simulink model "DB_HFI_sim"  (R2017a)
settings: Solver=ode45  StartTime=0.0  StopTime=20  FixedStep=0.5e-4  MaxStep=1e-4  RelTol=2.8e-10  AbsTol=eps  EnableMultiTasking=on
InitFcn:
  | %makec
model workspace: external: MAT-File C:\Users\Bench_39\Documents\MATLAB\DBDTFC_SelfSensing\ws.mat (data not in the file)
values from neighbouring files (symbols this model uses):
  bp = 2.2e-4    (= 0.00022)    [IPMSM_param.m]    (also in ws.mat)
  j = [0, -1; 1, 0]    [init.m]    (also in ws.mat = [0  -1; 1  0])
  Jp = 3.2e-4    (= 0.00032)    [IPMSM_param.m]    (also in ws.mat)
  lambda_pm = 0.13    [IPMSM_param.m]    (also in ws.mat)
  Ld = 8e-3    (= 0.008)    [IPMSM_param.m]    (also in ws.mat)
  Ldq = [Ld Lqd ;  Lqd Lq]    [IPMSM_param.m]    (also in ws.mat = [0.008  0; 0  0.02])
  Lq = 20e-3    (= 0.02)    [IPMSM_param.m]    (also in ws.mat)
  p = 2    [IPMSM_param.m]    (also in ws.mat)
  Rs = 1.35    [IPMSM_param.m]    (also in ws.mat)
  Ts = 1/fs    (= 0.0001)    [IPMSM_param.m]    (also in ws.mat)
undefined symbols (not defined in the file or in its folder): tau
libraries: plecslib_extras2 x2
settings Model: PauseTimes=1.11  ParamWorkspaceSource=ReferencedWorkspace  ExtModeTrigDuration=100  Creator=marc  LastModifiedBy=Gene
settings SolverCC: ConsecutiveZCsStepRelTol=eps  ZeroCrossControl=EnableAll
settings DataIOCC: ExternalInput=getinputstruct(op)  InitialState=getstatestruct(op)  SaveFormat=StructureWithTime  SaveOutput=off  SignalLogging=off  DSMLogging=off  VisualizeSimOutput=off  SaveTime=off  StateSaveName=tmp_raccel_xout  TimeSaveName=time  OutputSaveName=tmp_raccel_yout1,tmp_raccel_yout2  SignalLoggingName=tmp_raccel_logsout
settings OptimizationCC: DefaultParameterBehavior=Inlined  EfficientMapNaN2IntZero=off  LifeSpan=inf
settings DebuggingCC: AlgebraicLoopMsg=none  UnderspecifiedInitializationDetection=Classic  MergeDetectMultiDrivingBlocksExec=none  VectorMatrixConversionMsg=warning  UnconnectedInputMsg=none  UnconnectedOutputMsg=none  UnconnectedLineMsg=none  AllowSymbolicDim=off  StateNameClashWarn=warning  SFUnexpectedBacktrackingDiag=warning  SFNoUnconditionalDefaultTransitionDiag=warning  SFExecutionAtInitializationDiag=none
settings HardwareCC: ProdBitPerPointer=32  ProdBitPerSizeT=32  ProdBitPerPtrDiffT=32  ProdLargestAtomicFloat=None  ProdIntDivRoundTo=Undefined  ProdEndianess=Unspecified  ProdWordSize=32  ProdHWDeviceType=32-bit Generic  TargetBitPerPointer=64  TargetBitPerSizeT=64  TargetBitPerPtrDiffT=64  TargetLongLongMode=on  TargetIntDivRoundTo=Zero  TargetEndianess=LittleEndian  TargetWordSize=64  TargetHWDeviceType=MATLAB Host  ProdEqTarget=off
settings ModelReferenceCC: ParallelModelReferenceMATLABWorkerInit=Copy Base Workspace  PropagateSignalLabelsOutOfModel=off
settings RTWCC: SystemTargetFile=raccel.tlc  TemplateMakefile=raccel_default_tmf  RTWVerbose=off  RTWUseSimCustomCode=on
settings CodeAppCC: GenerateComments=off  MaxIdLength=128  MangleLength=10  SimulinkBlockComments=off
settings RaccelTargetCC: GeneratePreprocessorConditionals=Disable all  ERTFirstTimeCompliant=off  MultiInstanceERTCode=off  ENABLE_SLEXEC_SSBRIDGE=0  RTWCAPIParams=off
settings ConfigComp: CovMetricSettings=dw  CovHtmlReporting=on  CovSaveCumulativeToWorkspaceVar=on  CovSaveSingleToWorkspaceVar=on  CovExternalEMLEnable=off  CovSFcnEnable=off

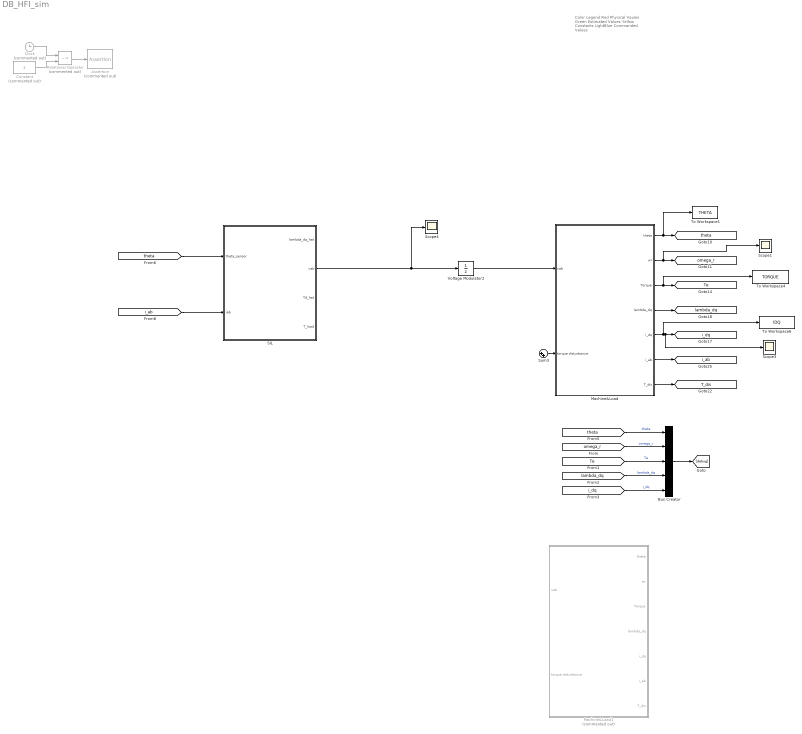
== system DB_HFI_sim ==
  note: Color Legend
      | Red Physical Vaules
      | Green Estimated Values
      | Yellow Constants
      | LightBlue Commanded Values
  Assertion : Assertion  Commented=on  AssertionFailFcn=|  StopWhenAssertionFail=off  SampleTime=Ts
      | set_param(bdroot,'SimulationCommand','pause'),
      | disp(sprintf('\nSimulation paused.'))
  Bus Creator : BusCreator  Inputs=5
  Clock : Clock  Commented=on
  Constant : Constant  Commented=on  SampleTime=Ts
  Machine&Load : Subsystem  TreatAsAtomicUnit=on
      settings: MinAlgLoopOccurrences=on
  Machine&Load1 : Subsystem  Commented=on  TreatAsAtomicUnit=on  SystemSampleTime=Ts
  Relational Operator : RelationalOperator  Commented=on  Operator=~=  OutDataTypeStr=boolean  RndMeth=Nearest
  SIL : Subsystem  TreatAsAtomicUnit=on  SystemSampleTime=Ts
  Scope1 : Scope
  Scope3 : Scope
  Scope4 : Scope
  Sum3 : Sum  Inputs=|++
  To Workspace1 : ToWorkspace  VariableName=THETA  SaveFormat=Structure With Time  SampleTime=Ts
  To Workspace4 : ToWorkspace  VariableName=TORQUE  SaveFormat=Structure With Time  SampleTime=Ts
  To Workspace6 : ToWorkspace  VariableName=IDQ  SaveFormat=Structure With Time  SampleTime=Ts
  Voltage Modulator2 : UnitDelay  InitialCondition=[0 0]  SampleTime=Ts
  tag scope: T_dis=global, Te=global, i_ab=global, i_dq=global, lambda_dq=global, omega_r=global, theta=global
  wires:
  Clock/1 -> Relational Operator/1
  Constant/1 -> Relational Operator/2
  Relational Operator/1 -> Assertion/1
  Machine&Load/1(theta) -> To Workspace1/1, [theta]
  Machine&Load/2(wr) -> Scope1/1, [omega_r]
  Machine&Load/3(Torque) -> To Workspace4/1, [Te]
  Machine&Load/4(lambda_dq) -> [lambda_dq]
  Machine&Load/5(i_dq) -> To Workspace6/1, Scope3/1, [i_dq]
  Machine&Load/7(T_dis) -> [T_dis]
  Machine&Load/6(i_ab) -> [i_ab]
  Bus Creator/1 -> [debug]
  [i_dq] -> Bus Creator/5  "i_dq"
  [lambda_dq] -> Bus Creator/4  "lambda_dq"
  [Te] -> Bus Creator/3  "Te"
  [omega_r] -> Bus Creator/2  "omega_r"
  [theta] -> Bus Creator/1  "theta"
  [i_ab] -> SIL/2(iab)
  Voltage Modulator2/1 -> Machine&Load/1(vab)
  Sum3/1 -> Machine&Load/2(torque disturbance)
  [theta] -> SIL/1(theta_sensor)
  SIL/2(vab) -> Scope4/1, Voltage Modulator2/1

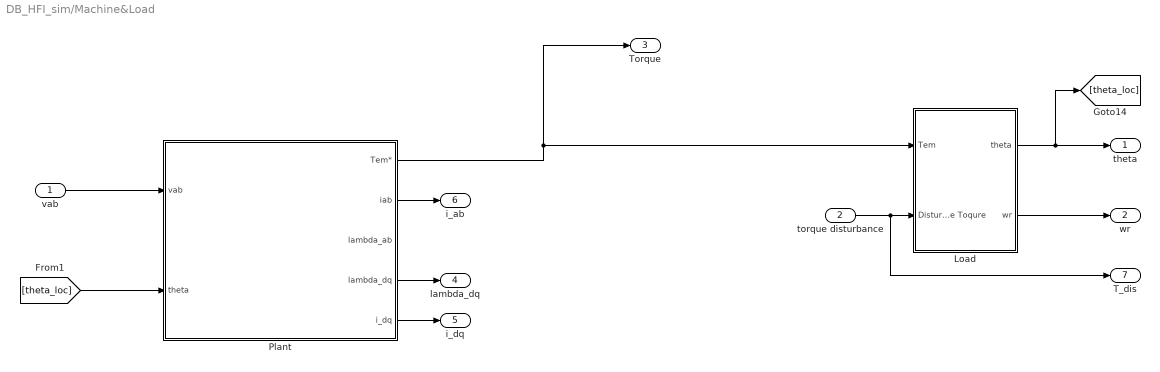
== system DB_HFI_sim/Machine&Load ==
  vab : Inport
  torque disturbance : Inport  Port=2
  Load : Subsystem
  Plant : Subsystem
  theta : Outport
  wr : Outport  Port=2
  Torque : Outport  Port=3
  lambda_dq : Outport  Port=4
  i_dq : Outport  Port=5
  i_ab : Outport  Port=6
  T_dis : Outport  Port=7
  wires:
  Load/2(wr) -> wr/1
  torque disturbance/1 -> T_dis/1, Load/2(Disturbance Toqure)
  Plant/4(lambda_dq) -> lambda_dq/1
  Plant/5(i_dq) -> i_dq/1
  vab/1 -> Plant/1(vab)
  Plant/2(iab) -> i_ab/1
  Load/1(theta) -> theta/1, [theta_loc]
  [theta_loc] -> Plant/2(theta)
  Plant/1(Tem*) -> Load/1(Tem), Torque/1

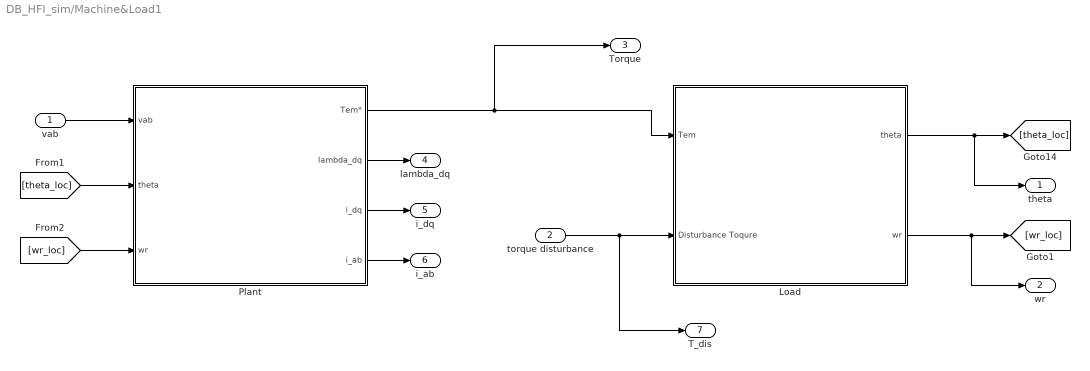
== system DB_HFI_sim/Machine&Load1 ==
  vab : Inport
  torque disturbance : Inport  Port=2
  Load : Subsystem
  Plant : Subsystem
  theta : Outport
  wr : Outport  Port=2
  Torque : Outport  Port=3
  lambda_dq : Outport  Port=4
  i_dq : Outport  Port=5
  i_ab : Outport  Port=6
  T_dis : Outport  Port=7
  wires:
  Load/1(theta) -> theta/1, [theta_loc]
  Load/2(wr) -> wr/1, [wr_loc]
  torque disturbance/1 -> T_dis/1, Load/2(Disturbance Toqure)
  Plant/1(Tem*) -> Load/1(Tem), Torque/1
  [theta_loc] -> Plant/2(theta)
  Plant/2(lambda_dq) -> lambda_dq/1
  Plant/3(i_dq) -> i_dq/1
  vab/1 -> Plant/1(vab)
  Plant/4(i_ab) -> i_ab/1
  [wr_loc] -> Plant/3(wr)

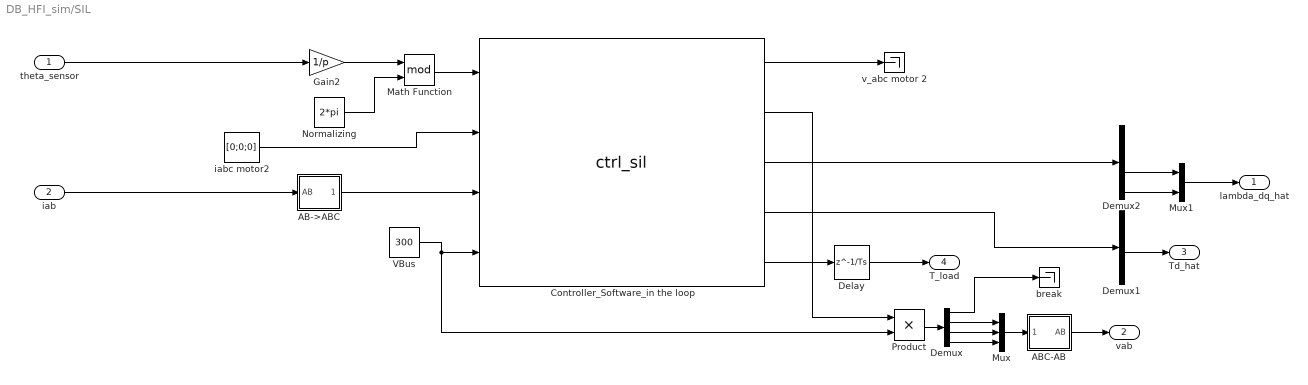
== system DB_HFI_sim/SIL ==
  theta_sensor : Inport
  iab : Inport  Port=2
  AB->ABC : Subsystem
  ABC-AB : Subsystem
  Controller_Software_in the loop : S-Function  FunctionName=ctrl_sil  Parameters=wr_set, T_com_set, lambda_com_set  SFunctionDeploymentMode=off  EnableBusSupport=off  mask{wr_set=20, T_com_set=0, lambda_com_set=lambda_pm}
      mask prompts: wr_set "Speed"; T_com_set "Torque"; lambda_com_set "Flux"
      mask Display:
      | image('governor.png')
      | port_label('output', 1, 'v_abc_motor2');
      | port_label('output', 2, 'v_abc_motor1');
      | port_label('output', 3, 'Current & Flux');
      | port_label('output', 4, 'debug');
      | port_label('output', 5, 'T_load');
  Delay : Delay  DelayLength=1/Ts
  Demux : Demux
  Demux1 : Demux  Outputs=6
  Demux2 : Demux
  Gain2 : Gain  Gain=1/p
  Math Function : Math  Operator=mod  SampleTime=Ts  SaturateOnIntegerOverflow=on
  Mux : Mux  Inputs=3
  Mux1 : Mux  Inputs=2
  Normalizing : Constant  Value=2*pi  SampleTime=Ts
  Product : Product
  VBus : Constant  Value=300  SampleTime=Ts
  break : Terminator
  iabc motor2 : Constant  Value=[0;0;0]  SampleTime=Ts
  v_abc motor 2 : Terminator
  lambda_dq_hat : Outport
  vab : Outport  Port=2
  Td_hat : Outport  Port=3
  T_load : Outport  Port=4
  wires:
  theta_sensor/1 -> Gain2/1
  Controller_Software_in the loop/2 -> Product/1
  VBus/1 -> Product/2, Controller_Software_in the loop/4
  AB->ABC/1(ABC) -> Controller_Software_in the loop/3
  Normalizing/1 -> Math Function/2
  Math Function/1 -> Controller_Software_in the loop/1
  Controller_Software_in the loop/4 -> Demux1/1
  Controller_Software_in the loop/1 -> v_abc motor 2/1
  iab/1 -> AB->ABC/1(AB)
  iabc motor2/1 -> Controller_Software_in the loop/2
  Gain2/1 -> Math Function/1
  Demux/2 -> Mux/1
  Demux/3 -> Mux/2
  Demux/4 -> Mux/3
  Demux/1 -> break/1
  Product/1 -> Demux/1
  Controller_Software_in the loop/5 -> Delay/1
  Delay/1 -> T_load/1
  Demux1/4 -> Td_hat/1
  Controller_Software_in the loop/3 -> Demux2/1
  Demux2/4 -> Mux1/2
  Demux2/3 -> Mux1/1
  Mux1/1 -> lambda_dq_hat/1
  Mux/1 -> ABC-AB/1(ABC)
  ABC-AB/1(AB) -> vab/1

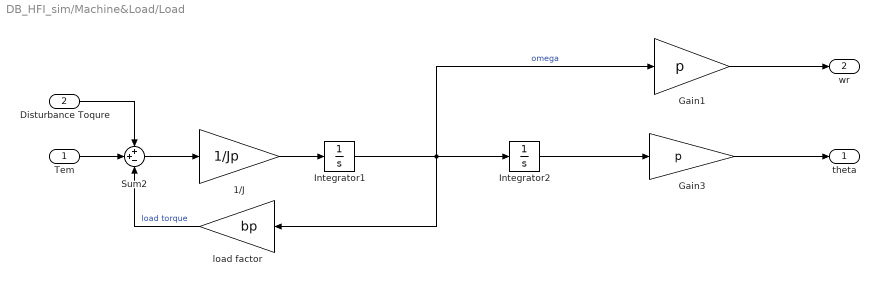
== system DB_HFI_sim/Machine&Load/Load ==
  Tem : Inport
  Disturbance Toqure : Inport  Port=2
  1/J : Gain  Gain=1/Jp
  Gain1 : Gain  Gain=p
  Gain3 : Gain  Gain=p
  Integrator1 : Integrator
  Integrator2 : Integrator
  Sum2 : Sum  Inputs=++-
  load factor : Gain  Gain=bp
  theta : Outport
  wr : Outport  Port=2
  wires:
  Gain1/1 -> wr/1
  Gain3/1 -> theta/1
  Sum2/1 -> 1/J/1
  1/J/1 -> Integrator1/1
  Integrator2/1 -> Gain3/1
  Tem/1 -> Sum2/2
  Disturbance Toqure/1 -> Sum2/1
  Integrator1/1 -> Integrator2/1, Gain1/1, load factor/1  "omega"
  load factor/1 -> Sum2/3  "load torque"

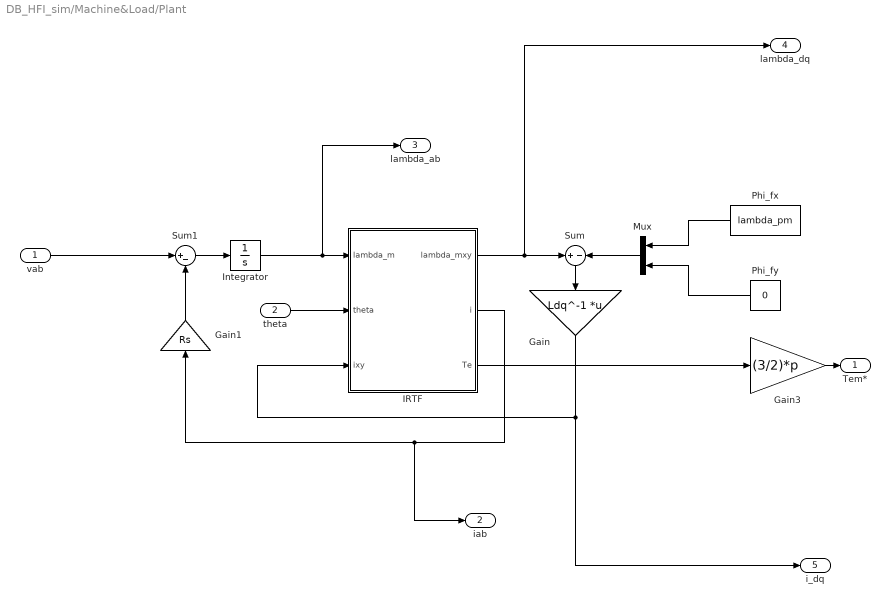
== system DB_HFI_sim/Machine&Load/Plant ==
  vab : Inport
  theta : Inport  Port=2
  Gain : Gain  Gain=Ldq^-1  Multiplication=Matrix(K*u) (u vector)
  Gain1 : Gain  Gain=Rs
  Gain3 : Gain  Gain=(3/2)*p
  IRTF : Subsystem
  Integrator : Integrator  InitialCondition=[lambda_pm;0]
  Mux : Mux  Inputs=2
  Phi_fx : Constant  Value=lambda_pm
  Phi_fy : Constant  Value=0
  Sum : Sum  Inputs=+|-
  Sum1 : Sum  Inputs=|+-
  Tem* : Outport
  iab : Outport  Port=2
  lambda_ab : Outport  Port=3
  lambda_dq : Outport  Port=4
  i_dq : Outport  Port=5
  wires:
  Integrator/1 -> lambda_ab/1, IRTF/1(lambda_m)
  IRTF/2(i) -> iab/1, Gain1/1
  Sum1/1 -> Integrator/1
  Sum/1 -> Gain/1
  Phi_fy/1 -> Mux/2
  Phi_fx/1 -> Mux/1
  IRTF/3(Te) -> Gain3/1
  Gain/1 -> i_dq/1, IRTF/3(ixy)
  IRTF/1(lambda_mxy) -> lambda_dq/1, Sum/1
  vab/1 -> Sum1/1
  Gain3/1 -> Tem*/1
  theta/1 -> IRTF/2(theta)
  Mux/1 -> Sum/2
  Gain1/1 -> Sum1/2

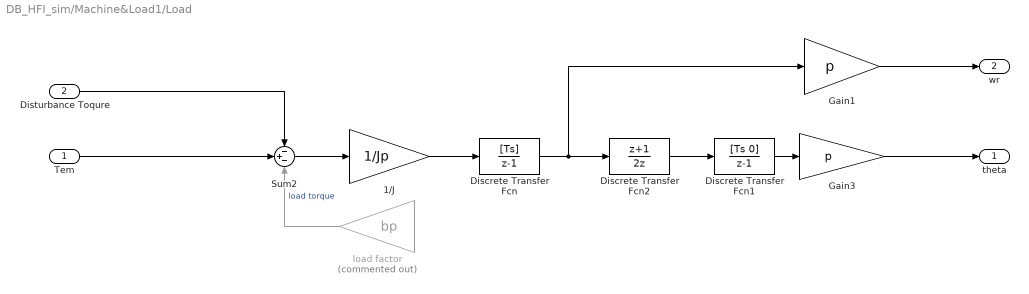
== system DB_HFI_sim/Machine&Load1/Load ==
  Tem : Inport
  Disturbance Toqure : Inport  Port=2
  1/J : Gain  Gain=1/Jp
  Discrete Transfer Fcn : DiscreteTransferFcn  Numerator=[Ts]  Denominator=[1 -1]  SampleTime=Ts
  Discrete Transfer Fcn1 : DiscreteTransferFcn  Numerator=[Ts 0]  Denominator=[1 -1]
  Discrete Transfer Fcn2 : DiscreteTransferFcn  Numerator=[1 1]  Denominator=[2 0]
  Gain1 : Gain  Gain=p
  Gain3 : Gain  Gain=p
  Sum2 : Sum  Inputs=-+-
  load factor : Gain  Commented=on  Gain=bp
  theta : Outport
  wr : Outport  Port=2
  wires:
  Gain1/1 -> wr/1
  Gain3/1 -> theta/1
  Sum2/1 -> 1/J/1
  1/J/1 -> Discrete Transfer Fcn/1
  Tem/1 -> Sum2/2
  Disturbance Toqure/1 -> Sum2/1
  load factor/1 -> Sum2/3  "load torque"
  Discrete Transfer Fcn/1 -> Gain1/1, Discrete Transfer Fcn2/1
  Discrete Transfer Fcn2/1 -> Discrete Transfer Fcn1/1
  Discrete Transfer Fcn1/1 -> Gain3/1

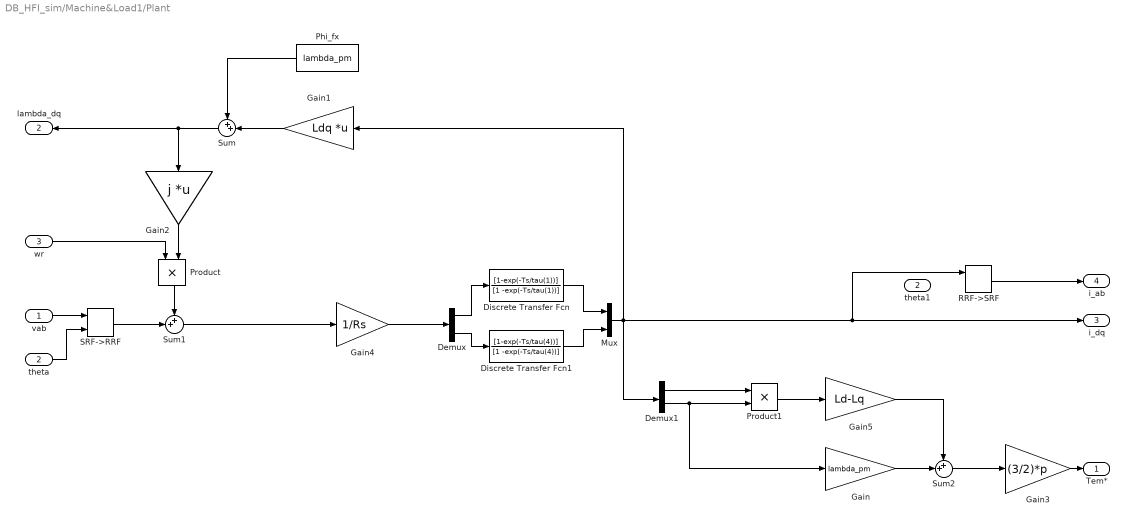
== system DB_HFI_sim/Machine&Load1/Plant ==
  vab : Inport
  theta : Inport  Port=2
  wr : Inport  Port=3
  Demux : Demux  Outputs=2
  Demux1 : Demux  Outputs=2
  Discrete Transfer Fcn : DiscreteTransferFcn  Numerator=[1-exp(-Ts/tau(1))]  Denominator=[1 -exp(-Ts/tau(1))]  SampleTime=Ts
  Discrete Transfer Fcn1 : DiscreteTransferFcn  Numerator=[1-exp(-Ts/tau(4))]  Denominator=[1 -exp(-Ts/tau(4))]  SampleTime=Ts
  Gain : Gain  Gain=lambda_pm
  Gain1 : Gain  Gain=Ldq  Multiplication=Matrix(K*u) (u vector)
  Gain2 : Gain  Gain=j  Multiplication=Matrix(K*u) (u vector)
  Gain3 : Gain  Gain=(3/2)*p
  Gain4 : Gain  Gain=1/Rs
  Gain5 : Gain  Gain=Ld-Lq
  Mux : Mux  Inputs=2
  Phi_fx : Constant  Value=lambda_pm  SampleTime=Ts
  Product : Product
  Product1 : Product
  RRF->SRF : plecslib_extras2/Transformations/RRF->SRF
  SRF->RRF : plecslib_extras2/Transformations/SRF->RRF
  Sum : Sum  Inputs=++|
  Sum1 : Sum  Inputs=++|
  Sum2 : Sum  Inputs=++|
  theta1 : InportShadow  Port=2
  Tem* : Outport
  lambda_dq : Outport  Port=2
  i_dq : Outport  Port=3
  i_ab : Outport  Port=4
  wires:
  Gain3/1 -> Tem*/1
  Gain4/1 -> Demux/1
  Demux/1 -> Discrete Transfer Fcn/1
  Demux/2 -> Discrete Transfer Fcn1/1
  Discrete Transfer Fcn/1 -> Mux/1
  Discrete Transfer Fcn1/1 -> Mux/2
  Gain1/1 -> Sum/2
  Phi_fx/1 -> Sum/1
  Mux/1 -> Demux1/1, RRF->SRF/1, i_dq/1, Gain1/1
  Sum1/1 -> Gain4/1
  SRF->RRF/1 -> Sum1/2
  vab/1 -> SRF->RRF/1
  theta/1 -> SRF->RRF/2
  Sum/1 -> Gain2/1, lambda_dq/1
  Gain2/1 -> Product/2
  wr/1 -> Product/1
  Demux1/1 -> Product1/1
  Demux1/2 -> Gain/1, Product1/2
  Product1/1 -> Gain5/1
  Gain/1 -> Sum2/2
  Gain5/1 -> Sum2/1
  Sum2/1 -> Gain3/1
  RRF->SRF/1 -> i_ab/1
  Product/1 -> Sum1/1

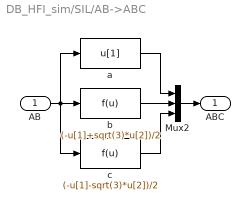
== system DB_HFI_sim/SIL/AB->ABC ==
  AB : Inport
  Mux2 : Mux  Inputs=3
  a : Fcn  Expr=u[1]
  b : Fcn  Expr=(-u[1]+sqrt(3)*u[2])/2
  c : Fcn  Expr=(-u[1]-sqrt(3)*u[2])/2
  ABC : Outport
  wires:
  Mux2/1 -> ABC/1
  b/1 -> Mux2/2
  c/1 -> Mux2/3
  AB/1 -> b/1, a/1, c/1
  a/1 -> Mux2/1

== system DB_HFI_sim/SIL/ABC-AB ==
  ABC : Inport
  Mux2 : Mux  Inputs=2
  a : Fcn  Expr=2/3*(u[1] -0.5*u[2] - 0.5*u[3])
  b : Fcn  Expr=2/3*(0 +sqrt(3)/2*u[2] - sqrt(3)/2*u[3])
  AB : Outport
  wires:
  Mux2/1 -> AB/1
  b/1 -> Mux2/2
  ABC/1 -> b/1, a/1
  a/1 -> Mux2/1

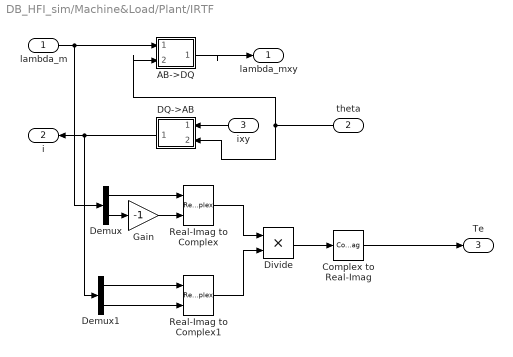
== system DB_HFI_sim/Machine&Load/Plant/IRTF ==
  lambda_m : Inport
  theta : Inport  Port=2
  ixy : Inport  Port=3
  AB->DQ : Subsystem
  Complex to Real-Imag : ComplexToRealImag  Output=Imag
  DQ->AB : Subsystem
  Demux : Demux  Outputs=2
  Demux1 : Demux  Outputs=2
  Divide : Product  Inputs=**
  Gain : Gain  Gain=-1
  Real-Imag to Complex : RealImagToComplex
  Real-Imag to Complex1 : RealImagToComplex
  lambda_mxy : Outport
  i : Outport  Port=2
  Te : Outport  Port=3
  wires:
  lambda_m/1 -> AB->DQ/1(AB), Demux/1
  AB->DQ/1(DQ) -> lambda_mxy/1
  theta/1 -> DQ->AB/2(Phi), AB->DQ/2(Phi)
  Complex to Real-Imag/1 -> Te/1
  Demux/1 -> Real-Imag to Complex/1
  Demux/2 -> Gain/1
  DQ->AB/1(AB) -> Demux1/1, i/1
  Demux1/1 -> Real-Imag to Complex1/1
  Demux1/2 -> Real-Imag to Complex1/2
  Gain/1 -> Real-Imag to Complex/2
  Real-Imag to Complex/1 -> Divide/1
  Real-Imag to Complex1/1 -> Divide/2
  Divide/1 -> Complex to Real-Imag/1
  ixy/1 -> DQ->AB/1(DQ)

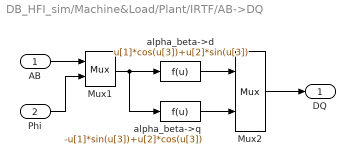
== system DB_HFI_sim/Machine&Load/Plant/IRTF/AB->DQ ==
  AB : Inport
  Phi : Inport  Port=2
  Mux1 : Mux  Inputs=2
  Mux2 : Mux  Inputs=2
  alpha_beta->d : Fcn  Expr=u[1]*cos(u[3])+u[2]*sin(u[3])
  alpha_beta->q : Fcn  Expr=-u[1]*sin(u[3])+u[2]*cos(u[3])
  DQ : Outport
  wires:
  Phi/1 -> Mux1/2
  AB/1 -> Mux1/1
  alpha_beta->q/1 -> Mux2/2
  alpha_beta->d/1 -> Mux2/1
  Mux2/1 -> DQ/1
  Mux1/1 -> alpha_beta->d/1, alpha_beta->q/1

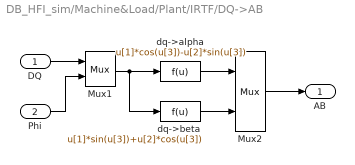
== system DB_HFI_sim/Machine&Load/Plant/IRTF/DQ->AB ==
  DQ : Inport
  Phi : Inport  Port=2
  Mux1 : Mux  Inputs=2
  Mux2 : Mux  Inputs=2
  dq->alpha : Fcn  Expr=u[1]*cos(u[3])-u[2]*sin(u[3])
  dq->beta : Fcn  Expr=u[1]*sin(u[3])+u[2]*cos(u[3])
  AB : Outport
  wires:
  Mux1/1 -> dq->alpha/1, dq->beta/1
  Mux2/1 -> AB/1
  dq->beta/1 -> Mux2/2
  dq->alpha/1 -> Mux2/1
  Phi/1 -> Mux1/2
  DQ/1 -> Mux1/1
